simulink model "One_Phase_SPWM_Inverter"  (R2015a)
settings: Solver=ode45  StartTime=0.0  StopTime=2  RelTol=1e-3
libraries: powerlib x9, powerlib_meascontrol x2, simulink x1
settings Model: Creator=Koustubh  LastModifiedBy=Koustubh

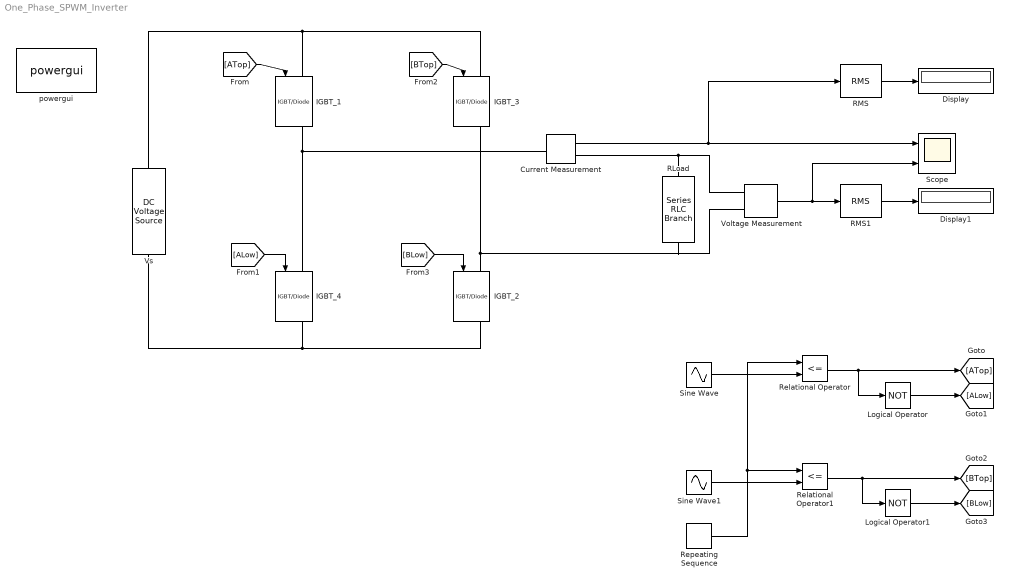
== system One_Phase_SPWM_Inverter ==
  Current Measurement : powerlib/Measurements/Current Measurement  PhasorSimulation=off  OutputType=Complex  PSBequivalent=0
  Display : Display
  Display1 : Display
  IGBT_{1..4} (4 alike) : powerlib/Power Electronics/IGBT//Diode  Ron=1e-3  Rs=1e5  Cs=inf  Measurements=on
  Logical Operator : Logic  Operator=NOT  AllPortsSameDT=off  OutDataTypeStr=boolean
  Logical Operator1 : Logic  Operator=NOT  AllPortsSameDT=off  OutDataTypeStr=boolean
  RLoad : powerlib/Elements/Series RLC Branch  LConnTagsString=__new0  RConnTagsString=__new0  BranchType=R  Resistance=10  Inductance=1e-3  SetiL0=off  InitialCurrent=0  Capacitance=1e-6  Setx0=off  InitialVoltage=0  Measurements=None
  RMS : powerlib_meascontrol/Measurements/RMS  TrueRMS=on  Freq=60  RMSInit=120  Ts=0
  RMS1 : powerlib_meascontrol/Measurements/RMS  TrueRMS=on  Freq=60  RMSInit=120  Ts=0
  Relational Operator : RelationalOperator  Operator=<=  OutDataTypeStr=boolean
  Relational Operator1 : RelationalOperator  Operator=<=  OutDataTypeStr=boolean
  Repeating Sequence : simulink/Sources/Repeating Sequence  rep_seq_t=[0 0.005 0.01]  rep_seq_y=[-1 1 -1]
  Scope : Scope  NumInputPorts=2
      settings: YMin=-5~-5  YMax=5~5
  Sine Wave : Sin  Frequency=2*pi*50  SampleTime=0
  Sine Wave1 : Sin  Frequency=2*pi*50  Phase=pi  SampleTime=0
  Voltage Measurement : powerlib/Measurements/Voltage Measurement  PhasorSimulation=off  OutputType=Complex  PSBequivalent=0
  Vs : powerlib/Electrical Sources/DC Voltage Source  Amplitude=230  Measurements=None
  powergui : powerlib/powergui  Priority=1  SimulationMode=Discrete  SolverType=Tustin/Backward Euler (TBE)  SampleTime=50e-6  frequency=60  SPID=off  DisableSnubberDevices=off  DisableRonSwitches=off  DisableVfSwitches=off  SwTol=0  DisplayEquations=off  Interpol=off  methode=off  Ts=100  FunctionMessages=off  echomessages=off  HookPort=off  EnableUseOfTLC=off  x0status=blocks  frequencyindice=0  Pbase=100e6  ErrMax=1e-4  Iterations=50  UnitsV=kV  UnitsW=MW  buscounter=0  RestoreLinks=warning  ResistiveCurrentMeasurement=off  Frange=[0:2:500]  Ylog=off  Xlog=on  ShowGrid=off  save=off  variable=ZData  structure=0  ZoomFFT=off  StartTime=0.0  cycles=1  DisplayStyle=1  fundamental=60  FreqAxis=off  MaxFrequency=1000  frequencyindicesteady=1  RmsSteady=1  display=off
  wires:
  Sine Wave/1 -> Relational Operator/2
  Repeating Sequence/1 -> Relational Operator1/1, Relational Operator/1
  Sine Wave1/1 -> Relational Operator1/2
  Relational Operator/1 -> Logical Operator/1, [ATop]
  Logical Operator/1 -> [ALow]
  Relational Operator1/1 -> Logical Operator1/1, [BTop]
  Logical Operator1/1 -> [BLow]
  [ATop] -> IGBT_1/1
  [BLow] -> IGBT_2/1
  [BTop] -> IGBT_3/1
  [ALow] -> IGBT_4/1
  Current Measurement/1 -> Scope/1, RMS/1
  Voltage Measurement/1 -> RMS1/1, Scope/2
  RMS/1 -> Display/1
  RMS1/1 -> Display1/1
  connections:
  IGBT_3/RConn1 -- Voltage Measurement/LConn2 -- RLoad/RConn1 -- IGBT_2/LConn1
  IGBT_1/RConn1 -- IGBT_4/LConn1 -- Current Measurement/LConn1
  IGBT_1/LConn1 -- IGBT_3/LConn1 -- Vs/RConn1
  IGBT_4/RConn1 -- IGBT_2/RConn1 -- Vs/LConn1
  RLoad/LConn1 -- Current Measurement/RConn1 -- Voltage Measurement/LConn1
